simulink model "DR18E_Testpult"  (R2017a)
settings: Solver=ode1  StartTime=0.0  StopTime=Inf  FixedStep=0.001  RelTol=1e-3
PostLoadFcn:
  | , if any(exist('dsrtsu_mdlpostloadfcn', 'file') == [2, 3, 6]), try dsrtsu_mdlpostloadfcn('Execute', bdroot); catch fprintf('Error in PostLoadFcn (dsrtsu_mdlpostloadfcn) for model "%s":\n %s\n', bdroot, lasterr); end, end,
model workspace: external: MAT-File C:\Users\DeltaRacing\Documents\dSPACE\MABX_DR18E\Model\DR18E_MABX_Parameter.mat (data not in the file)
values from neighbouring files (symbols this model uses):
  am = 1/Ts    (= 1)    [DR18E_MABX_Parameter.m]
  bm = K/Ts    (= 0.05)    [DR18E_MABX_Parameter.m]
  cf = 41350    [DR18E_MABX_Parameter.m]
  cr = 41350    [DR18E_MABX_Parameter.m]
  Derating_HV_Battery_Kapa = 1    [DR18E_MABX_Parameter.m]
  Derating_Start_km = 16    [DR18E_MABX_Parameter.m]
  Drive_Mode = 0    [DR18E_MABX_Parameter.m]
  g = 1    [DR18E_MABX_Parameter.m]
  Gas_Modus = 2    [DR18E_MABX_Parameter.m]
  HV_Power_max = 80    [DR18E_MABX_Parameter.m]
  i_Getriebe = 3.3    [DR18E_MABX_Parameter.m]
  i_Lenkgetriebe = 4.32    [DR18E_MABX_Parameter.m]
  K_SET = 1    [DR18E_MABX_Parameter.m]
  Kapazitaet_HV_Battery_kWh = 6.6    [DR18E_MABX_Parameter.m]
  KW_T_Soll = 37    [DR18E_MABX_Parameter.m]
  lf = 1.2    [DR18E_MABX_Parameter.m]
  lr = 1.15    [DR18E_MABX_Parameter.m]
  m = mdriver + mvehicle    (= 310)    [DR18E_MABX_Parameter.m]
  M_max = 150    [DR18E_MABX_Parameter.m]
  Power_Limit_onoff = 0    [DR18E_MABX_Parameter.m]
  Reifenradius = 0.2351    [DR18E_MABX_Parameter.m]
  Strecke_Endu_km = 22    [DR18E_MABX_Parameter.m]
  TC_Decr_Gas = 0.00005    (= 5e-05)    [DR18E_MABX_Parameter.m]
  TC_Derivative = 0.4    [DR18E_MABX_Parameter.m]
  TC_Incr_Gas = 0.005    [DR18E_MABX_Parameter.m]
  TC_On = 0    [DR18E_MABX_Parameter.m]
  TC_Relay_Off = 0.065    [DR18E_MABX_Parameter.m]
  TC_Relay_On = 0.07    [DR18E_MABX_Parameter.m]
  TV_Mode = 2    [DR18E_MABX_Parameter.m]
  TV_On = 0    [DR18E_MABX_Parameter.m]
  TV_Override = 1    [DR18E_MABX_Parameter.m]
  y = 0.8    [DR18E_MABX_Parameter.m]
undefined symbols (not defined in the file or in its folder): D, DiscIntNeverNeededParam, I, K_OL, P
libraries: simulink x288, rtican x100, rtiusbflightreclib x40, rti1401lib_dio_type3 x10, simulink_extras x10, rti1401lib_adc_type4 x8, rti1401lib_II_base x7
(part 23 of 27)

== system DR18E_Testpult/Eingabe Fahrzeug/BMS/Voltage Stack 7-8/Voltage Stack 8 ==
  Timeout[samples] : Inport
  Bus Creator : BusCreator  Inputs=12
  HV_STK8A : rtican/RTICAN Receive (RX)   Reserved1=[]  Reserved2=[]  Reserved3=[]  Reserved4=[]  SfcnMessage=[]  Msg_Struct=[]  BoardTypeNo=[]  BoardNo=[]  ChannelNo=[]  Parameters=[]  DialogFcn=[]  UnitName=[]  Revision=[]  UnitValues=[]  DSProperties=struct('RTI',struct('Version',uint32(5),'BlockType',struct('isSLSource',uint8(1),'isSLSink',uint8(1),'isHWSource',uint8(0),'isHWSink',uint8(0),'isSetup',uint8(0),'isInline',uint8(1),'isNonInline',uint8(0),'isInterrupt',uint8(0),'isChannelwise',uint8(0)),'IOBoardType','RTICAN','UnitType','MESSAGE','Identifier','RX','DialogType','MSVC','BlockSet','RTICAN','SlaveProcessor','CAN'))  RTIBlockInterface=struct('OutputPortsWidth',int32([1 1 1 1 1 1 1]),'OutputPortsActive',[1 1 1 1 1 1 1],'OutputPortsName',{{'Cell_Voltage_85','Cell_Voltage_86','Cell_Voltage_87','Cell_Voltage_88',['RX status'],['RX time'],['RX delta time']}},'OutputPortsDataType',{{'SS_DOUBLE','SS_DOUBLE','SS_DOUBLE','SS_DOUBLE','SS_DOUBLE','SS_DOUBLE','SS_DOUBLE'}},'OutputPortsLabel',{{'Cell_Voltage_85','Cell_Voltage_86','Cell_Voltage_87','Cell_Voltage_88','','',''}},'OutputPortsLabelMode','ON','InputPortsWidth',int32(0),'InputPortsActive',0,'DialogFcn','rtican_message_interface_gui','BlockDisplay',{{'','center'}},'IconTransparency','on','ParameterTunableNames',{{}},'InitLevel',3,'BlockName',struct('Token',{{'HV_STK8A'}}),'SampleTime',{{-1}},'TriggerPort',{{'none'}},'EnablePort',{{'none'}})  RTIBlockParameters=struct('BoardTypeNo',{{1,'OFF',[]}},'BoardNo',{{2,'ON',[1 16]}},'ChannelNo',{{1,'ON',[1 2]}},'Parameters',{{struct('DataFileSupport',struct('DataFileSelectedMaster',1,'DataFileSelectedLocal',1,'DataFileName','c:\users\deltaracing\documents\canoe\dr18e\dbc\dr18e.dbc|','DataFileDate',['16-Feb-2019 13:23:09'],'SelectedFile','..\..\..\canoe\dr18e_test\dr18e\dbc\dr18e.dbc','InterfaceFcn','rtican_dbc_file_parser'),'Options',struct('StatusSelected',1,'TimeSelected',1,'DeltaTimeSelected',1,'BytePortSelected',0,'MessageLengthSelected',0,'TriggerPort',struct('Selected',0,'TriggerType',0),'UserCoding',struct('Selected',0,'InterfaceFile','UserDecodingFile','FcnName','UserDecodeFcn','InportSelected',0,'InportWidth',1,'OutportSelected',0,'OutportWidth',1),'EnablePortSelected',0,'SignalOnPortnameSelected',1,'UseRXService',0),'Message',struct('MsgOnBlocknameSelected',1,'MsgName','HV_STK8A','MsgIdFormat',0,'MsgId',357,'MsgLength',8,'NumSignals',4,'SampleTime',-1,'Signal',struct('SgnName',{'Cell_Voltage_85','Cell_Voltage_86','Cell_Voltage_87','Cell_Voltage_88'},'SgnStartBit',{0,16,32,48},'SgnLength',{16,16,16,16},'ByteLayout',{0,0,0,0},'Factor',{0.001,0.001,0.001,0.001},'Offset',{0,0,0,0},'SgnComment',{'','','',''},'SgnUnit',{'V','V','V','V'},'Min',{0,0,0,0},'Max',{0,0,0,0},'SgnType',{0,0,0,0},'SLDataType',{'SS_DOUBLE','SS_DOUBLE','SS_DOUBLE','SS_DOUBLE'},'DataType',{0,0,0,0},'ModeValue',{-1,-1,-1,-1}),'MsgIdNumFormat',0,'MsgComment',{{''}}),'Version',1.2,'general',struct('isFromLib',0)),'OFF',[]}},'GroupId',{{struct('Group',{{'RTICAN'}},'No',1,'Behavior',{{'NAMECHANGE'}},'BlockType',{{'SINK'}},'NameChangeFlag',0),'OFF',[]}},'SFcnRTICANMessage',{{struct('MsgType','RX','SFcnPortType','Scalar','MsgName','HV_STK8A','MsgIdFormat','STD','MsgId',357,'MsgLength',8,'NumSignals',4,'SampleTime',-1,'Signal',struct('SgnName',{'Cell_Voltage_85','Cell_Voltage_86','Cell_Voltage_87','Cell_Voltage_88'},'SgnStartBit',{0,16,32,48},'SgnLength',{16,16,16,16},'ByteLayout',{['little endian'],['little endian'],['little endian'],['little endian']},'Factor',{0.001,0.001,0.001,0.001},'Offset',{0,0,0,0},'SgnType',{'standard','standard','standard','standard'},'SLDataType',{'SS_DOUBLE','SS_DOUBLE','SS_DOUBLE','SS_DOUBLE'},'DataType',{['unsigned int'],['unsigned int'],['unsigned int'],['unsigned int']},'ModeValue',{-1,-1,-1,-1}),'StatusSelected','yes','TimeSelected','yes','DeltaTimeSelected','yes','BytePortSelected','no','MessageLengthSelected','no','TriggerPort',struct('Selected','no','TriggerType',0),'UserCoding',struct('Selected','no','InterfaceFile','UserDecodingFile','FcnName','UserDecodeFcn','InportSelected','no','InportWidth',1,'OutportSelected','no','OutportWidth',1),'EnablePortSelected','no','UseRXService','no','BoardType','DS1','BoardNo',2,'ControllerNo',1),'OFF',[]}},'TLCFileName',{{'rtican_rx_message','OFF',[]}})  RTISFcnParameters=struct('SFcnRTICANMessage','struct','TLCFileName','char')  RTIBlockParaDefault=struct('BoardTypeNo',4302,'BoardNo',1,'ChannelNo',1,'Parameters',struct('DataFileSupport',struct('DataFileSelectedMaster',0,'DataFileSelectedLocal',0,'DataFileName','','DataFileDate','','SelectedFile',['<no file selected>']),'Options',struct('StatusSelected',1,'TimeSelected',1,'DeltaTimeSelected',1,'BytePortSelected',0,'MessageLengthSelected',0,'TriggerPort',struct('Selected',0,'TriggerType','rising'),'UserCoding',struct('Selected',0,'InterfaceFile','UserDecodingFile','FcnName','UserDecodeFcn','InportSelected',0,'InportWidth',1,'OutportSelected',0,'OutportWidth',1),'EnablePortSelected',0,'SignalOnPortnameSelected',1,'UseRXService',0),'Message',struct('MsgOnBlocknameSelected',0,'MsgName',['RX Message'],'MsgIdFormat',0,'MsgId',100,'MsgLength',8,'NumSignals',1,'SampleTime',-1,'Signal',struct('SgnName',['RX signal'],'SgnStartBit',0,'SgnLength',8,'SgnType',0,'ModeValue',-1,'DataType',0,'SLDataType','SS_DOUBLE','ByteLayout',0,'Factor',1,'Offset',0,'Min',0,'Max',255,'SgnComment',{{}},'SgnUnit',''),'MsgIdNumFormat',0,'MsgComment',{{''}}),'Version',1.2,'general',struct('isFromLib',1)),'GroupId',struct('Group',{{'RTICAN'}},'No',1,'Behavior',{{'NAMECHANGE'}},'BlockType',{{'SINK'}},'NameChangeFlag',0),'SFcnRTICANMessage',struct('MsgType','RX','MsgName',['RX Message'],'MsgIdFormat','STD','MsgId',100,'MsgLength',8,'NumSignals',1,'SampleTime',-1,'Signal',struct('SgnName',['RX signal'],'SgnStartBit',0,'SgnLength',8,'SgnType','standard','ModeValue',-1,'DataType',['unsigned int'],'ByteLayout',['little endian'],'SLDataType','SS_DOUBLE','Factor',1,'Offset',0),'StatusSelected','yes','TimeSelected','yes','DeltaTimeSelected','yes','BytePortSelected','no','MessageLengthSelected','no','EnablePortSelected','no','UserCoding',struct('Selected','no','InterfaceFile','UserDecodingFile','FcnName','UserDecodeFcn','InportSelected','no','InportWidth',1,'OutportSelected','no','OutportWidth',1),'TriggerPort',struct('Selected','no','TriggerType','rising'),'UseRXService','no','BoardType','DS4302','BoardNo',1,'ControllerNo',1,'SFcnPortType','Scalar'),'TLCFileName','rtican_rx_message')
      settings: AttributesFormatString=Group Id: RTICAN1\n  SourceProductName=dSPACE RTI CAN Blockset
  HV_STK8B : rtican/RTICAN Receive (RX)   Reserved1=[]  Reserved2=[]  Reserved3=[]  Reserved4=[]  SfcnMessage=[]  Msg_Struct=[]  BoardTypeNo=[]  BoardNo=[]  ChannelNo=[]  Parameters=[]  DialogFcn=[]  UnitName=[]  Revision=[]  UnitValues=[]  DSProperties=struct('RTI',struct('Version',uint32(5),'BlockType',struct('isSLSource',uint8(1),'isSLSink',uint8(1),'isHWSource',uint8(0),'isHWSink',uint8(0),'isSetup',uint8(0),'isInline',uint8(1),'isNonInline',uint8(0),'isInterrupt',uint8(0),'isChannelwise',uint8(0)),'IOBoardType','RTICAN','UnitType','MESSAGE','Identifier','RX','DialogType','MSVC','BlockSet','RTICAN','SlaveProcessor','CAN'))  RTIBlockInterface=struct('OutputPortsWidth',int32([1 1 1 1 1 1 1]),'OutputPortsActive',[1 1 1 1 1 1 1],'OutputPortsName',{{'Cell_Voltage_89','Cell_Voltage_90','Cell_Voltage_91','Cell_Voltage_92',['RX status'],['RX time'],['RX delta time']}},'OutputPortsDataType',{{'SS_DOUBLE','SS_DOUBLE','SS_DOUBLE','SS_DOUBLE','SS_DOUBLE','SS_DOUBLE','SS_DOUBLE'}},'OutputPortsLabel',{{'Cell_Voltage_89','Cell_Voltage_90','Cell_Voltage_91','Cell_Voltage_92','','',''}},'OutputPortsLabelMode','ON','InputPortsWidth',int32(0),'InputPortsActive',0,'DialogFcn','rtican_message_interface_gui','BlockDisplay',{{'','center'}},'IconTransparency','on','ParameterTunableNames',{{}},'InitLevel',3,'BlockName',struct('Token',{{'HV_STK8B'}}),'SampleTime',{{-1}},'TriggerPort',{{'none'}},'EnablePort',{{'none'}})  RTIBlockParameters=struct('BoardTypeNo',{{1,'OFF',[]}},'BoardNo',{{2,'ON',[1 16]}},'ChannelNo',{{1,'ON',[1 2]}},'Parameters',{{struct('DataFileSupport',struct('DataFileSelectedMaster',1,'DataFileSelectedLocal',1,'DataFileName','c:\users\deltaracing\documents\canoe\dr18e\dbc\dr18e.dbc|','DataFileDate',['16-Feb-2019 13:23:09'],'SelectedFile','..\..\..\canoe\dr18e_test\dr18e\dbc\dr18e.dbc','InterfaceFcn','rtican_dbc_file_parser'),'Options',struct('StatusSelected',1,'TimeSelected',1,'DeltaTimeSelected',1,'BytePortSelected',0,'MessageLengthSelected',0,'TriggerPort',struct('Selected',0,'TriggerType',0),'UserCoding',struct('Selected',0,'InterfaceFile','UserDecodingFile','FcnName','UserDecodeFcn','InportSelected',0,'InportWidth',1,'OutportSelected',0,'OutportWidth',1),'EnablePortSelected',0,'SignalOnPortnameSelected',1,'UseRXService',0),'Message',struct('MsgOnBlocknameSelected',1,'MsgName','HV_STK8B','MsgIdFormat',0,'MsgId',358,'MsgLength',8,'NumSignals',4,'SampleTime',-1,'Signal',struct('SgnName',{'Cell_Voltage_89','Cell_Voltage_90','Cell_Voltage_91','Cell_Voltage_92'},'SgnStartBit',{0,16,32,48},'SgnLength',{16,16,16,16},'ByteLayout',{0,0,0,0},'Factor',{0.001,0.001,0.001,0.001},'Offset',{0,0,0,0},'SgnComment',{'','','',''},'SgnUnit',{'V','V','V','V'},'Min',{0,0,0,0},'Max',{0,0,0,0},'SgnType',{0,0,0,0},'SLDataType',{'SS_DOUBLE','SS_DOUBLE','SS_DOUBLE','SS_DOUBLE'},'DataType',{0,0,0,0},'ModeValue',{-1,-1,-1,-1}),'MsgIdNumFormat',0,'MsgComment',{{''}}),'Version',1.2,'general',struct('isFromLib',0)),'OFF',[]}},'GroupId',{{struct('Group',{{'RTICAN'}},'No',1,'Behavior',{{'NAMECHANGE'}},'BlockType',{{'SINK'}},'NameChangeFlag',0),'OFF',[]}},'SFcnRTICANMessage',{{struct('MsgType','RX','SFcnPortType','Scalar','MsgName','HV_STK8B','MsgIdFormat','STD','MsgId',358,'MsgLength',8,'NumSignals',4,'SampleTime',-1,'Signal',struct('SgnName',{'Cell_Voltage_89','Cell_Voltage_90','Cell_Voltage_91','Cell_Voltage_92'},'SgnStartBit',{0,16,32,48},'SgnLength',{16,16,16,16},'ByteLayout',{['little endian'],['little endian'],['little endian'],['little endian']},'Factor',{0.001,0.001,0.001,0.001},'Offset',{0,0,0,0},'SgnType',{'standard','standard','standard','standard'},'SLDataType',{'SS_DOUBLE','SS_DOUBLE','SS_DOUBLE','SS_DOUBLE'},'DataType',{['unsigned int'],['unsigned int'],['unsigned int'],['unsigned int']},'ModeValue',{-1,-1,-1,-1}),'StatusSelected','yes','TimeSelected','yes','DeltaTimeSelected','yes','BytePortSelected','no','MessageLengthSelected','no','TriggerPort',struct('Selected','no','TriggerType',0),'UserCoding',struct('Selected','no','InterfaceFile','UserDecodingFile','FcnName','UserDecodeFcn','InportSelected','no','InportWidth',1,'OutportSelected','no','OutportWidth',1),'EnablePortSelected','no','UseRXService','no','BoardType','DS1','BoardNo',2,'ControllerNo',1),'OFF',[]}},'TLCFileName',{{'rtican_rx_message','OFF',[]}})  RTISFcnParameters=struct('SFcnRTICANMessage','struct','TLCFileName','char')  RTIBlockParaDefault=struct('BoardTypeNo',4302,'BoardNo',1,'ChannelNo',1,'Parameters',struct('DataFileSupport',struct('DataFileSelectedMaster',0,'DataFileSelectedLocal',0,'DataFileName','','DataFileDate','','SelectedFile',['<no file selected>']),'Options',struct('StatusSelected',1,'TimeSelected',1,'DeltaTimeSelected',1,'BytePortSelected',0,'MessageLengthSelected',0,'TriggerPort',struct('Selected',0,'TriggerType','rising'),'UserCoding',struct('Selected',0,'InterfaceFile','UserDecodingFile','FcnName','UserDecodeFcn','InportSelected',0,'InportWidth',1,'OutportSelected',0,'OutportWidth',1),'EnablePortSelected',0,'SignalOnPortnameSelected',1,'UseRXService',0),'Message',struct('MsgOnBlocknameSelected',0,'MsgName',['RX Message'],'MsgIdFormat',0,'MsgId',100,'MsgLength',8,'NumSignals',1,'SampleTime',-1,'Signal',struct('SgnName',['RX signal'],'SgnStartBit',0,'SgnLength',8,'SgnType',0,'ModeValue',-1,'DataType',0,'SLDataType','SS_DOUBLE','ByteLayout',0,'Factor',1,'Offset',0,'Min',0,'Max',255,'SgnComment',{{}},'SgnUnit',''),'MsgIdNumFormat',0,'MsgComment',{{''}}),'Version',1.2,'general',struct('isFromLib',1)),'GroupId',struct('Group',{{'RTICAN'}},'No',1,'Behavior',{{'NAMECHANGE'}},'BlockType',{{'SINK'}},'NameChangeFlag',0),'SFcnRTICANMessage',struct('MsgType','RX','MsgName',['RX Message'],'MsgIdFormat','STD','MsgId',100,'MsgLength',8,'NumSignals',1,'SampleTime',-1,'Signal',struct('SgnName',['RX signal'],'SgnStartBit',0,'SgnLength',8,'SgnType','standard','ModeValue',-1,'DataType',['unsigned int'],'ByteLayout',['little endian'],'SLDataType','SS_DOUBLE','Factor',1,'Offset',0),'StatusSelected','yes','TimeSelected','yes','DeltaTimeSelected','yes','BytePortSelected','no','MessageLengthSelected','no','EnablePortSelected','no','UserCoding',struct('Selected','no','InterfaceFile','UserDecodingFile','FcnName','UserDecodeFcn','InportSelected','no','InportWidth',1,'OutportSelected','no','OutportWidth',1),'TriggerPort',struct('Selected','no','TriggerType','rising'),'UseRXService','no','BoardType','DS4302','BoardNo',1,'ControllerNo',1,'SFcnPortType','Scalar'),'TLCFileName','rtican_rx_message')
      settings: AttributesFormatString=Group Id: RTICAN1\n  SourceProductName=dSPACE RTI CAN Blockset
  HV_STK8C : rtican/RTICAN Receive (RX)   Reserved1=[]  Reserved2=[]  Reserved3=[]  Reserved4=[]  SfcnMessage=[]  Msg_Struct=[]  BoardTypeNo=[]  BoardNo=[]  ChannelNo=[]  Parameters=[]  DialogFcn=[]  UnitName=[]  Revision=[]  UnitValues=[]  DSProperties=struct('RTI',struct('Version',uint32(5),'BlockType',struct('isSLSource',uint8(1),'isSLSink',uint8(1),'isHWSource',uint8(0),'isHWSink',uint8(0),'isSetup',uint8(0),'isInline',uint8(1),'isNonInline',uint8(0),'isInterrupt',uint8(0),'isChannelwise',uint8(0)),'IOBoardType','RTICAN','UnitType','MESSAGE','Identifier','RX','DialogType','MSVC','BlockSet','RTICAN','SlaveProcessor','CAN'))  RTIBlockInterface=struct('OutputPortsWidth',int32([1 1 1 1 1 1 1]),'OutputPortsActive',[1 1 1 1 1 1 1],'OutputPortsName',{{'Cell_Voltage_93','Cell_Voltage_94','Cell_Voltage_95','Cell_Voltage_96',['RX status'],['RX time'],['RX delta time']}},'OutputPortsDataType',{{'SS_DOUBLE','SS_DOUBLE','SS_DOUBLE','SS_DOUBLE','SS_DOUBLE','SS_DOUBLE','SS_DOUBLE'}},'OutputPortsLabel',{{'Cell_Voltage_93','Cell_Voltage_94','Cell_Voltage_95','Cell_Voltage_96','','',''}},'OutputPortsLabelMode','ON','InputPortsWidth',int32(0),'InputPortsActive',0,'DialogFcn','rtican_message_interface_gui','BlockDisplay',{{'','center'}},'IconTransparency','on','ParameterTunableNames',{{}},'InitLevel',3,'BlockName',struct('Token',{{'HV_STK8C'}}),'SampleTime',{{-1}},'TriggerPort',{{'none'}},'EnablePort',{{'none'}})  RTIBlockParameters=struct('BoardTypeNo',{{1,'OFF',[]}},'BoardNo',{{2,'ON',[1 16]}},'ChannelNo',{{1,'ON',[1 2]}},'Parameters',{{struct('DataFileSupport',struct('DataFileSelectedMaster',1,'DataFileSelectedLocal',1,'DataFileName','c:\users\deltaracing\documents\canoe\dr18e\dbc\dr18e.dbc|','DataFileDate',['16-Feb-2019 13:23:09'],'SelectedFile','..\..\..\canoe\dr18e_test\dr18e\dbc\dr18e.dbc','InterfaceFcn','rtican_dbc_file_parser'),'Options',struct('StatusSelected',1,'TimeSelected',1,'DeltaTimeSelected',1,'BytePortSelected',0,'MessageLengthSelected',0,'TriggerPort',struct('Selected',0,'TriggerType',0),'UserCoding',struct('Selected',0,'InterfaceFile','UserDecodingFile','FcnName','UserDecodeFcn','InportSelected',0,'InportWidth',1,'OutportSelected',0,'OutportWidth',1),'EnablePortSelected',0,'SignalOnPortnameSelected',1,'UseRXService',0),'Message',struct('MsgOnBlocknameSelected',1,'MsgName','HV_STK8C','MsgIdFormat',0,'MsgId',359,'MsgLength',8,'NumSignals',4,'SampleTime',-1,'Signal',struct('SgnName',{'Cell_Voltage_93','Cell_Voltage_94','Cell_Voltage_95','Cell_Voltage_96'},'SgnStartBit',{0,16,32,48},'SgnLength',{16,16,16,16},'ByteLayout',{0,0,0,0},'Factor',{0.001,0.001,0.001,0.001},'Offset',{0,0,0,0},'SgnComment',{'','','',''},'SgnUnit',{'V','V','V','V'},'Min',{0,0,0,0},'Max',{0,0,0,0},'SgnType',{0,0,0,0},'SLDataType',{'SS_DOUBLE','SS_DOUBLE','SS_DOUBLE','SS_DOUBLE'},'DataType',{0,0,0,0},'ModeValue',{-1,-1,-1,-1}),'MsgIdNumFormat',0,'MsgComment',{{''}}),'Version',1.2,'general',struct('isFromLib',0)),'OFF',[]}},'GroupId',{{struct('Group',{{'RTICAN'}},'No',1,'Behavior',{{'NAMECHANGE'}},'BlockType',{{'SINK'}},'NameChangeFlag',0),'OFF',[]}},'SFcnRTICANMessage',{{struct('MsgType','RX','SFcnPortType','Scalar','MsgName','HV_STK8C','MsgIdFormat','STD','MsgId',359,'MsgLength',8,'NumSignals',4,'SampleTime',-1,'Signal',struct('SgnName',{'Cell_Voltage_93','Cell_Voltage_94','Cell_Voltage_95','Cell_Voltage_96'},'SgnStartBit',{0,16,32,48},'SgnLength',{16,16,16,16},'ByteLayout',{['little endian'],['little endian'],['little endian'],['little endian']},'Factor',{0.001,0.001,0.001,0.001},'Offset',{0,0,0,0},'SgnType',{'standard','standard','standard','standard'},'SLDataType',{'SS_DOUBLE','SS_DOUBLE','SS_DOUBLE','SS_DOUBLE'},'DataType',{['unsigned int'],['unsigned int'],['unsigned int'],['unsigned int']},'ModeValue',{-1,-1,-1,-1}),'StatusSelected','yes','TimeSelected','yes','DeltaTimeSelected','yes','BytePortSelected','no','MessageLengthSelected','no','TriggerPort',struct('Selected','no','TriggerType',0),'UserCoding',struct('Selected','no','InterfaceFile','UserDecodingFile','FcnName','UserDecodeFcn','InportSelected','no','InportWidth',1,'OutportSelected','no','OutportWidth',1),'EnablePortSelected','no','UseRXService','no','BoardType','DS1','BoardNo',2,'ControllerNo',1),'OFF',[]}},'TLCFileName',{{'rtican_rx_message','OFF',[]}})  RTISFcnParameters=struct('SFcnRTICANMessage','struct','TLCFileName','char')  RTIBlockParaDefault=struct('BoardTypeNo',4302,'BoardNo',1,'ChannelNo',1,'Parameters',struct('DataFileSupport',struct('DataFileSelectedMaster',0,'DataFileSelectedLocal',0,'DataFileName','','DataFileDate','','SelectedFile',['<no file selected>']),'Options',struct('StatusSelected',1,'TimeSelected',1,'DeltaTimeSelected',1,'BytePortSelected',0,'MessageLengthSelected',0,'TriggerPort',struct('Selected',0,'TriggerType','rising'),'UserCoding',struct('Selected',0,'InterfaceFile','UserDecodingFile','FcnName','UserDecodeFcn','InportSelected',0,'InportWidth',1,'OutportSelected',0,'OutportWidth',1),'EnablePortSelected',0,'SignalOnPortnameSelected',1,'UseRXService',0),'Message',struct('MsgOnBlocknameSelected',0,'MsgName',['RX Message'],'MsgIdFormat',0,'MsgId',100,'MsgLength',8,'NumSignals',1,'SampleTime',-1,'Signal',struct('SgnName',['RX signal'],'SgnStartBit',0,'SgnLength',8,'SgnType',0,'ModeValue',-1,'DataType',0,'SLDataType','SS_DOUBLE','ByteLayout',0,'Factor',1,'Offset',0,'Min',0,'Max',255,'SgnComment',{{}},'SgnUnit',''),'MsgIdNumFormat',0,'MsgComment',{{''}}),'Version',1.2,'general',struct('isFromLib',1)),'GroupId',struct('Group',{{'RTICAN'}},'No',1,'Behavior',{{'NAMECHANGE'}},'BlockType',{{'SINK'}},'NameChangeFlag',0),'SFcnRTICANMessage',struct('MsgType','RX','MsgName',['RX Message'],'MsgIdFormat','STD','MsgId',100,'MsgLength',8,'NumSignals',1,'SampleTime',-1,'Signal',struct('SgnName',['RX signal'],'SgnStartBit',0,'SgnLength',8,'SgnType','standard','ModeValue',-1,'DataType',['unsigned int'],'ByteLayout',['little endian'],'SLDataType','SS_DOUBLE','Factor',1,'Offset',0),'StatusSelected','yes','TimeSelected','yes','DeltaTimeSelected','yes','BytePortSelected','no','MessageLengthSelected','no','EnablePortSelected','no','UserCoding',struct('Selected','no','InterfaceFile','UserDecodingFile','FcnName','UserDecodeFcn','InportSelected','no','InportWidth',1,'OutportSelected','no','OutportWidth',1),'TriggerPort',struct('Selected','no','TriggerType','rising'),'UseRXService','no','BoardType','DS4302','BoardNo',1,'ControllerNo',1,'SFcnPortType','Scalar'),'TLCFileName','rtican_rx_message')
      settings: AttributesFormatString=Group Id: RTICAN1\n  SourceProductName=dSPACE RTI CAN Blockset
  Logical Operator : Logic  Operator=OR  Inputs=3  AllPortsSameDT=off  OutDataTypeStr=boolean
  RX Timeout Detection : Subsystem
  RX Timeout Detection1 : Subsystem
  RX Timeout Detection2 : Subsystem
  Cell73-84 : Outport
  TimeoutError : Outport  Port=2
  wires:
  HV_STK8B/5 -> RX Timeout Detection/1(RX status)
  HV_STK8C/5 -> RX Timeout Detection2/1(RX status)
  Bus Creator/1 -> Cell73-84/1  "Cell73-84"
  HV_STK8A/5 -> RX Timeout Detection1/1(RX status)
  RX Timeout Detection2/1(RX Timeout Error) -> Logical Operator/3
  RX Timeout Detection/1(RX Timeout Error) -> Logical Operator/2  "RX Timeout Error"
  RX Timeout Detection1/1(RX Timeout Error) -> Logical Operator/1
  Logical Operator/1 -> TimeoutError/1
  Timeout[samples]/1 -> RX Timeout Detection1/2(Timeout (n Samples)), RX Timeout Detection/2(Timeout (n Samples)), RX Timeout Detection2/2(Timeout (n Samples))
  HV_STK8A/1 -> Bus Creator/1  "Cell_Voltage_85"
  HV_STK8A/2 -> Bus Creator/2  "Cell_Voltage_86"
  HV_STK8A/3 -> Bus Creator/3  "Cell_Voltage_87"
  HV_STK8A/4 -> Bus Creator/4  "Cell_Voltage_88"
  HV_STK8B/1 -> Bus Creator/5  "Cell_Voltage_89"
  HV_STK8B/2 -> Bus Creator/6  "Cell_Voltage_90"
  HV_STK8B/3 -> Bus Creator/7  "Cell_Voltage_91"
  HV_STK8B/4 -> Bus Creator/8  "Cell_Voltage_92"
  HV_STK8C/1 -> Bus Creator/9  "Cell_Voltage_93"
  HV_STK8C/2 -> Bus Creator/10  "Cell_Voltage_94"
  HV_STK8C/3 -> Bus Creator/11  "Cell_Voltage_95"
  HV_STK8C/4 -> Bus Creator/12  "Cell_Voltage_96"

== system DR18E_Testpult/Eingabe Fahrzeug/Gyro/RX Timeout Detection/Triggered Subsystem ==
  TXStatus : Inport
  Timeout : Inport  Port=2
  Constant : Constant
  Constant1 : Constant  Value=0
  Constant2 : Constant
  Constant3 : Constant  Value=0
  Delay : Delay  DelayLength=1  InitialCondition=0
  Relational Operator : RelationalOperator  Operator=>  OutDataTypeStr=boolean  RndMeth=Nearest
  Sum : Sum  Inputs=|++
  Switch : Switch  Criteria=u2 > Threshold
  Switch1 : Switch  Criteria=u2 > Threshold
  Rampe : Outport
  RX Timeout Error : Outport  Port=2
  wires:
  TXStatus/1 -> Switch/2
  Delay/1 -> Sum/2
  Constant/1 -> Sum/1
  Sum/1 -> Switch/3
  Switch/1 -> Delay/1, Relational Operator/1, Rampe/1
  Constant1/1 -> Switch/1
  Constant2/1 -> Switch1/1
  Constant3/1 -> Switch1/3
  Switch1/1 -> RX Timeout Error/1
  Relational Operator/1 -> Switch1/2
  Timeout/1 -> Relational Operator/2

== system DR18E_Testpult/Eingabe Fahrzeug/Inverter Feedback Messages/Istwerte Umrichter 1 empfangen /Drehzahl ==
  CAN Value : Inport
  M_Mot : Inport  Port=2
  Action Port : ActionPort  ActionType=case
  2*pi / 60 : Gain  Gain=1.8*6.283185 / 60
  Constant1 : Constant
  Data Type Conversion : DataTypeConversion  OutDataTypeStr=int16
  Data Type Conversion1 : DataTypeConversion  OutDataTypeStr=double
  PT1 Discrete2 : Subsystem
  Product : Product
  Skalierung Drehzahl : Subsystem  TreatAsAtomicUnit=on
  TFilterDrehzahl : Constant  Value=0.01
  Drehzahl in 1/min U1 : Outport
  Motorleistung in W U1 : Outport  Port=2
  wires:
  CAN Value/1 -> Data Type Conversion/1
  Skalierung Drehzahl/1(Out1) -> PT1 Discrete2/1(u)
  Data Type Conversion/1 -> Data Type Conversion1/1
  Product/1 -> 2*pi / 60/1
  M_Mot/1 -> Product/2
  2*pi / 60/1 -> Motorleistung in W U1/1
  Constant1/1 -> PT1 Discrete2/2(K)
  TFilterDrehzahl/1 -> PT1 Discrete2/3(T)
  PT1 Discrete2/1(y) -> Drehzahl in 1/min U1/1, Product/1
  Data Type Conversion1/1 -> Skalierung Drehzahl/1(In1)

== system DR18E_Testpult/Eingabe Fahrzeug/Inverter Feedback Messages/Istwerte Umrichter 1 empfangen /FlightRecorder1 ==
  In1 : Inport
  Data Type Conversion : DataTypeConversion
  Gain : Gain
  USB_FLIGHT_REC_BL1 : rtiusbflightreclib/USB_FLIGHT_REC_BL1  VarName=UDC_HV  DataType=Single  SampleTime=-1  TLCFileName=rtiusbflightrecwrite  Reserved1=[]  Reserved2=[]  Reserved3=[]  Reserved4=[]  DSProperties=struct('RTI',struct('Version',uint32(3),'BlockType',struct('isSLSource',uint8(0),'isSLSink',uint8(1),'isHWSource',uint8(0),'isHWSink',uint8(0),'isSetup',uint8(0),'isInline',uint8(1),'isNonInline',uint8(0),'isInterrupt',uint8(0),'isChannelwise',uint8(0)),'IOBoardType',{{'DSUSB','FLIGHTREC'}},'UnitType','FLIGHTREC','Identifier','WRITE','DialogType','SL','BlockSet','RTIUSBFLIGHTREC','SlaveProcessor','NONE'))  RTIBlockInterface=struct('InputPortsActive',1,'InputPortsWidth',int32(1),'InputPortsDataType',{{'SS_SINGLE'}},'BlockDisplay',{{['Write to\nUSB Flight Recorder'],'center'}},'IconTransparency','off','InitLevel',3,'BlockName',struct('Token',{{'USB_FLIGHT_REC_BL1'}}),'MaskDescription',['Write input to the Flight Recorder. Recorded data can be referenced by the specified variable.'],'SampleTime',{{-1}})  RTIBlockParameters=struct('VarName',{{'UDC_HV','OFF',[]}},'DataType',{{'Single','OFF',[]}},'SampleTime',{{-1,'OFF',[]}},'TLCFileName',{{'rtiusbflightrecwrite','OFF',[]}})  RTISFcnParameters=struct('VarName','char','DataType','char','SampleTime','double','TLCFileName','char')  RTIBlockParaDefault=struct('VarName','Var1','DataType','Single','SampleTime',-1,'TLCFileName','rtiusbflightrecwrite')
      settings: SourceProductName=dSPACE RTI USB Flight Rec Blockset
  wires:
  Data Type Conversion/1 -> USB_FLIGHT_REC_BL1/1
  In1/1 -> Gain/1
  Gain/1 -> Data Type Conversion/1

== system DR18E_Testpult/Eingabe Fahrzeug/Inverter Feedback Messages/Istwerte Umrichter 1 empfangen /FlightRecorder2 ==
  In1 : Inport
  Data Type Conversion : DataTypeConversion
  Gain : Gain
  USB_FLIGHT_REC_BL1 : rtiusbflightreclib/USB_FLIGHT_REC_BL1  VarName=Inverter1Temp  DataType=Single  SampleTime=-1  TLCFileName=rtiusbflightrecwrite  Reserved1=[]  Reserved2=[]  Reserved3=[]  Reserved4=[]  DSProperties=struct('RTI',struct('Version',uint32(3),'BlockType',struct('isSLSource',uint8(0),'isSLSink',uint8(1),'isHWSource',uint8(0),'isHWSink',uint8(0),'isSetup',uint8(0),'isInline',uint8(1),'isNonInline',uint8(0),'isInterrupt',uint8(0),'isChannelwise',uint8(0)),'IOBoardType',{{'DSUSB','FLIGHTREC'}},'UnitType','FLIGHTREC','Identifier','WRITE','DialogType','SL','BlockSet','RTIUSBFLIGHTREC','SlaveProcessor','NONE'))  RTIBlockInterface=struct('InputPortsActive',1,'InputPortsWidth',int32(1),'InputPortsDataType',{{'SS_SINGLE'}},'BlockDisplay',{{['Write to\nUSB Flight Recorder'],'center'}},'IconTransparency','off','InitLevel',3,'BlockName',struct('Token',{{'USB_FLIGHT_REC_BL1'}}),'MaskDescription',['Write input to the Flight Recorder. Recorded data can be referenced by the specified variable.'],'SampleTime',{{-1}})  RTIBlockParameters=struct('VarName',{{'Inverter1Temp','OFF',[]}},'DataType',{{'Single','OFF',[]}},'SampleTime',{{-1,'OFF',[]}},'TLCFileName',{{'rtiusbflightrecwrite','OFF',[]}})  RTISFcnParameters=struct('VarName','char','DataType','char','SampleTime','double','TLCFileName','char')  RTIBlockParaDefault=struct('VarName','Var1','DataType','Single','SampleTime',-1,'TLCFileName','rtiusbflightrecwrite')
      settings: SourceProductName=dSPACE RTI USB Flight Rec Blockset
  wires:
  Data Type Conversion/1 -> USB_FLIGHT_REC_BL1/1
  In1/1 -> Gain/1
  Gain/1 -> Data Type Conversion/1

== system DR18E_Testpult/Eingabe Fahrzeug/Inverter Feedback Messages/Istwerte Umrichter 1 empfangen /FlightRecorder3 ==
  In1 : Inport
  Data Type Conversion : DataTypeConversion
  Gain : Gain
  USB_FLIGHT_REC_BL1 : rtiusbflightreclib/USB_FLIGHT_REC_BL1  VarName=MMotL_ist  DataType=Single  SampleTime=-1  TLCFileName=rtiusbflightrecwrite  Reserved1=[]  Reserved2=[]  Reserved3=[]  Reserved4=[]  DSProperties=struct('RTI',struct('Version',uint32(3),'BlockType',struct('isSLSource',uint8(0),'isSLSink',uint8(1),'isHWSource',uint8(0),'isHWSink',uint8(0),'isSetup',uint8(0),'isInline',uint8(1),'isNonInline',uint8(0),'isInterrupt',uint8(0),'isChannelwise',uint8(0)),'IOBoardType',{{'DSUSB','FLIGHTREC'}},'UnitType','FLIGHTREC','Identifier','WRITE','DialogType','SL','BlockSet','RTIUSBFLIGHTREC','SlaveProcessor','NONE'))  RTIBlockInterface=struct('InputPortsActive',1,'InputPortsWidth',int32(1),'InputPortsDataType',{{'SS_SINGLE'}},'BlockDisplay',{{['Write to\nUSB Flight Recorder'],'center'}},'IconTransparency','off','InitLevel',3,'BlockName',struct('Token',{{'USB_FLIGHT_REC_BL1'}}),'MaskDescription',['Write input to the Flight Recorder. Recorded data can be referenced by the specified variable.'],'SampleTime',{{-1}})  RTIBlockParameters=struct('VarName',{{'MMotL_ist','OFF',[]}},'DataType',{{'Single','OFF',[]}},'SampleTime',{{-1,'OFF',[]}},'TLCFileName',{{'rtiusbflightrecwrite','OFF',[]}})  RTISFcnParameters=struct('VarName','char','DataType','char','SampleTime','double','TLCFileName','char')  RTIBlockParaDefault=struct('VarName','Var1','DataType','Single','SampleTime',-1,'TLCFileName','rtiusbflightrecwrite')
      settings: SourceProductName=dSPACE RTI USB Flight Rec Blockset
  wires:
  Data Type Conversion/1 -> USB_FLIGHT_REC_BL1/1
  In1/1 -> Gain/1
  Gain/1 -> Data Type Conversion/1

== system DR18E_Testpult/Eingabe Fahrzeug/Inverter Feedback Messages/Istwerte Umrichter 1 empfangen /FlightRecorder4 ==
  In1 : Inport
  Data Type Conversion : DataTypeConversion
  Gain : Gain
  USB_FLIGHT_REC_BL1 : rtiusbflightreclib/USB_FLIGHT_REC_BL1  VarName=MotorLTemp  DataType=Single  SampleTime=-1  TLCFileName=rtiusbflightrecwrite  Reserved1=[]  Reserved2=[]  Reserved3=[]  Reserved4=[]  DSProperties=struct('RTI',struct('Version',uint32(3),'BlockType',struct('isSLSource',uint8(0),'isSLSink',uint8(1),'isHWSource',uint8(0),'isHWSink',uint8(0),'isSetup',uint8(0),'isInline',uint8(1),'isNonInline',uint8(0),'isInterrupt',uint8(0),'isChannelwise',uint8(0)),'IOBoardType',{{'DSUSB','FLIGHTREC'}},'UnitType','FLIGHTREC','Identifier','WRITE','DialogType','SL','BlockSet','RTIUSBFLIGHTREC','SlaveProcessor','NONE'))  RTIBlockInterface=struct('InputPortsActive',1,'InputPortsWidth',int32(1),'InputPortsDataType',{{'SS_SINGLE'}},'BlockDisplay',{{['Write to\nUSB Flight Recorder'],'center'}},'IconTransparency','off','InitLevel',3,'BlockName',struct('Token',{{'USB_FLIGHT_REC_BL1'}}),'MaskDescription',['Write input to the Flight Recorder. Recorded data can be referenced by the specified variable.'],'SampleTime',{{-1}})  RTIBlockParameters=struct('VarName',{{'MotorLTemp','OFF',[]}},'DataType',{{'Single','OFF',[]}},'SampleTime',{{-1,'OFF',[]}},'TLCFileName',{{'rtiusbflightrecwrite','OFF',[]}})  RTISFcnParameters=struct('VarName','char','DataType','char','SampleTime','double','TLCFileName','char')  RTIBlockParaDefault=struct('VarName','Var1','DataType','Single','SampleTime',-1,'TLCFileName','rtiusbflightrecwrite')
      settings: SourceProductName=dSPACE RTI USB Flight Rec Blockset
  wires:
  Data Type Conversion/1 -> USB_FLIGHT_REC_BL1/1
  In1/1 -> Gain/1
  Gain/1 -> Data Type Conversion/1

== system DR18E_Testpult/Eingabe Fahrzeug/Inverter Feedback Messages/Istwerte Umrichter 1 empfangen /Inverter_Temp ==
  In1 : Inport
  Action Port : ActionPort  ActionType=case
  "BAMOCAR PG D3 Manual S. 48 " : Lookup_n-D  NumberOfTableDimensions=1  BreakpointsForDimension1=[17151,17400,17688,18017,18387,18797,19247,19733,20250,20793,21357,21933,22515,23097,23671,24232,24775,25296,25792,26261,26702]  Table=[0,5,10,15,20,25,30,35,40,45,50,55,60,65,70,75,80,85,90,95,100]  RndMeth=Simplest  InputSameDT=on
  Inverter_Temp : Outport
  wires:
  In1/1 -> "BAMOCAR PG D3 Manual S. 48 "/1  "Wert"
  "BAMOCAR PG D3 Manual S. 48 "/1 -> Inverter_Temp/1

== system DR18E_Testpult/Eingabe Fahrzeug/Inverter Feedback Messages/Istwerte Umrichter 1 empfangen /Motortemperatur ==
  In1 : Inport
  Action Port : ActionPort  ActionType=case
  Constant2 : Constant  Value=37175
  Divide : Product  Inputs=*/
  Gain : Gain  Gain=4700
  Subtract : Sum  Inputs=+-
  Temp. corresponding resistance : Lookup_n-D  NumberOfTableDimensions=1  BreakpointsForDimension1=[1030,1135,1247,1367,1495,1630,1772,1922,2000,2080,2245,2417,2597,2785,2980,3182,3392,3607,3817,3915,4008,4166,4280]  IndexSearchMethod=Linear search  Table=[-50,-40,-30,-20,-10,0,10,20,25,30,40,50,60,70,80,90,100,110,120,125,130,140,150]  RndMeth=Simplest  InputSameDT=on
  Motor1_Temp : Outport
  "Motor1_Temp_Raw " : Outport  Port=2
  wires:
  Gain/1 -> Divide/1
  Subtract/1 -> Divide/2  "RawWert2_Motor1"
  Constant2/1 -> Subtract/1
  In1/1 -> Subtract/2, Gain/1  "Wert"
  Divide/1 -> "Motor1_Temp_Raw "/1, Temp. corresponding resistance/1
  Temp. corresponding resistance/1 -> Motor1_Temp/1

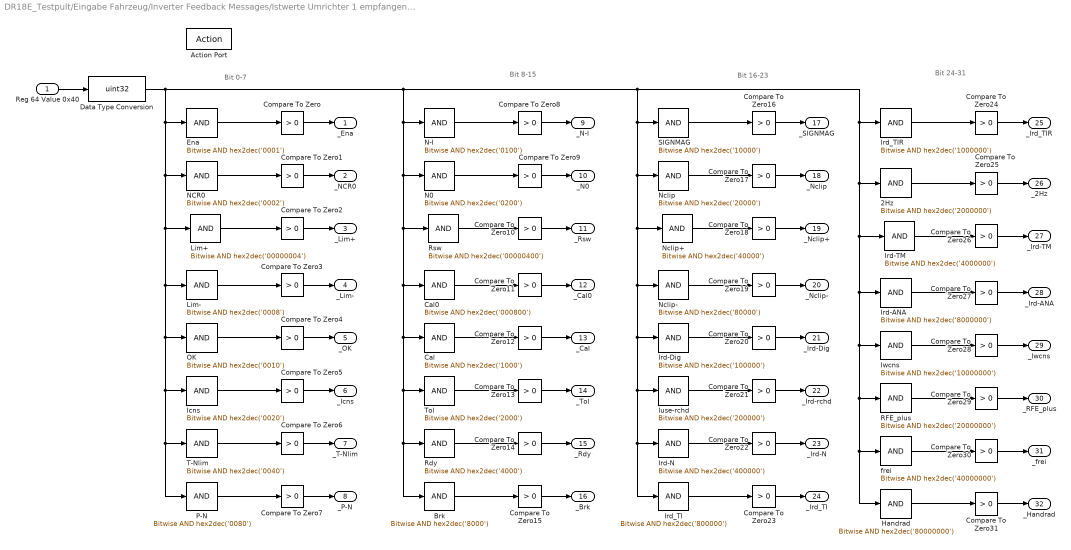
== system DR18E_Testpult/Eingabe Fahrzeug/Inverter Feedback Messages/Istwerte Umrichter 1 empfangen /Red ID 64: Status Register Auswertung ==
  note: Bit 24-31
  note: Bit 16-23
  note: Bit 8-15
  note: Bit 0-7
  Reg 64 Value 0x40 : Inport
  Action Port : ActionPort  ActionType=case
  2Hz : simulink/Logic and Bit Operations/Bitwise Operator  logicop=AND  UseBitMask=on  BitMask=hex2dec('2000000')  BitMaskRealWorld=Stored Integer
  Brk : simulink/Logic and Bit Operations/Bitwise Operator  logicop=AND  UseBitMask=on  BitMask=hex2dec('8000')  BitMaskRealWorld=Stored Integer
  Cal : simulink/Logic and Bit Operations/Bitwise Operator  logicop=AND  UseBitMask=on  BitMask=hex2dec('1000')  BitMaskRealWorld=Stored Integer
  Cal0 : simulink/Logic and Bit Operations/Bitwise Operator  logicop=AND  UseBitMask=on  BitMask=hex2dec('000800')  BitMaskRealWorld=Stored Integer
  Compare To Zero{,1..31} (32 alike) : simulink/Logic and Bit Operations/Compare To Zero  relop=>  OutDataTypeStr=boolean
  Data Type Conversion : DataTypeConversion  OutDataTypeStr=uint32
  Ena : simulink/Logic and Bit Operations/Bitwise Operator  logicop=AND  UseBitMask=on  BitMask=hex2dec('0001')  BitMaskRealWorld=Stored Integer
  Handrad : simulink/Logic and Bit Operations/Bitwise Operator  logicop=AND  UseBitMask=on  BitMask=hex2dec('80000000')  BitMaskRealWorld=Stored Integer
  Icns : simulink/Logic and Bit Operations/Bitwise Operator  logicop=AND  UseBitMask=on  BitMask=hex2dec('0020')  BitMaskRealWorld=Stored Integer
  Ird-ANA : simulink/Logic and Bit Operations/Bitwise Operator  logicop=AND  UseBitMask=on  BitMask=hex2dec('8000000')  BitMaskRealWorld=Stored Integer
  Ird-Dig : simulink/Logic and Bit Operations/Bitwise Operator  logicop=AND  UseBitMask=on  BitMask=hex2dec('100000')  BitMaskRealWorld=Stored Integer
  Ird-N : simulink/Logic and Bit Operations/Bitwise Operator  logicop=AND  UseBitMask=on  BitMask=hex2dec('400000')  BitMaskRealWorld=Stored Integer
  Ird-TM : simulink/Logic and Bit Operations/Bitwise Operator  logicop=AND  UseBitMask=on  BitMask=hex2dec('4000000')  BitMaskRealWorld=Stored Integer
  Ird_TI : simulink/Logic and Bit Operations/Bitwise Operator  logicop=AND  UseBitMask=on  BitMask=hex2dec('800000')  BitMaskRealWorld=Stored Integer
  Ird_TIR : simulink/Logic and Bit Operations/Bitwise Operator  logicop=AND  UseBitMask=on  BitMask=hex2dec('1000000')  BitMaskRealWorld=Stored Integer
  Iuse-rchd : simulink/Logic and Bit Operations/Bitwise Operator  logicop=AND  UseBitMask=on  BitMask=hex2dec('200000')  BitMaskRealWorld=Stored Integer
  Iwcns : simulink/Logic and Bit Operations/Bitwise Operator  logicop=AND  UseBitMask=on  BitMask=hex2dec('10000000')  BitMaskRealWorld=Stored Integer
  Lim+ : simulink/Logic and Bit Operations/Bitwise Operator  logicop=AND  UseBitMask=on  BitMask=hex2dec('00000004')  BitMaskRealWorld=Stored Integer
  Lim- : simulink/Logic and Bit Operations/Bitwise Operator  logicop=AND  UseBitMask=on  BitMask=hex2dec('0008')  BitMaskRealWorld=Stored Integer
  N-I : simulink/Logic and Bit Operations/Bitwise Operator  logicop=AND  UseBitMask=on  BitMask=hex2dec('0100')  BitMaskRealWorld=Stored Integer
  N0 : simulink/Logic and Bit Operations/Bitwise Operator  logicop=AND  UseBitMask=on  BitMask=hex2dec('0200')  BitMaskRealWorld=Stored Integer
  NCR0 : simulink/Logic and Bit Operations/Bitwise Operator  logicop=AND  UseBitMask=on  BitMask=hex2dec('0002')  BitMaskRealWorld=Stored Integer
  Nclip : simulink/Logic and Bit Operations/Bitwise Operator  logicop=AND  UseBitMask=on  BitMask=hex2dec('20000')  BitMaskRealWorld=Stored Integer
  Nclip+ : simulink/Logic and Bit Operations/Bitwise Operator  logicop=AND  UseBitMask=on  BitMask=hex2dec('40000')  BitMaskRealWorld=Stored Integer
  Nclip- : simulink/Logic and Bit Operations/Bitwise Operator  logicop=AND  UseBitMask=on  BitMask=hex2dec('80000')  BitMaskRealWorld=Stored Integer
  OK : simulink/Logic and Bit Operations/Bitwise Operator  logicop=AND  UseBitMask=on  BitMask=hex2dec('0010')  BitMaskRealWorld=Stored Integer
  P-N : simulink/Logic and Bit Operations/Bitwise Operator  logicop=AND  UseBitMask=on  BitMask=hex2dec('0080')  BitMaskRealWorld=Stored Integer
  RFE_plus : simulink/Logic and Bit Operations/Bitwise Operator  logicop=AND  UseBitMask=on  BitMask=hex2dec('20000000')  BitMaskRealWorld=Stored Integer
  Rdy : simulink/Logic and Bit Operations/Bitwise Operator  logicop=AND  UseBitMask=on  BitMask=hex2dec('4000')  BitMaskRealWorld=Stored Integer
  Rsw : simulink/Logic and Bit Operations/Bitwise Operator  logicop=AND  UseBitMask=on  BitMask=hex2dec('00000400')  BitMaskRealWorld=Stored Integer
  SIGNMAG : simulink/Logic and Bit Operations/Bitwise Operator  logicop=AND  UseBitMask=on  BitMask=hex2dec('10000')  BitMaskRealWorld=Stored Integer
  T-Nlim : simulink/Logic and Bit Operations/Bitwise Operator  logicop=AND  UseBitMask=on  BitMask=hex2dec('0040')  BitMaskRealWorld=Stored Integer
  Tol : simulink/Logic and Bit Operations/Bitwise Operator  logicop=AND  UseBitMask=on  BitMask=hex2dec('2000')  BitMaskRealWorld=Stored Integer
  frei : simulink/Logic and Bit Operations/Bitwise Operator  logicop=AND  UseBitMask=on  BitMask=hex2dec('40000000')  BitMaskRealWorld=Stored Integer
  _Ena : Outport
  _NCR0 : Outport  Port=2
  _Lim+ : Outport  Port=3
  _Lim- : Outport  Port=4
  _OK : Outport  Port=5
  _Icns : Outport  Port=6
  _T-Nlim : Outport  Port=7
  _P-N : Outport  Port=8
  _N-I : Outport  Port=9
  _N0 : Outport  Port=10
  _Rsw : Outport  Port=11
  _Cal0 : Outport  Port=12
  _Cal : Outport  Port=13
  _Tol : Outport  Port=14
  _Rdy : Outport  Port=15
  _Brk : Outport  Port=16
  _SIGNMAG : Outport  Port=17
  _Nclip : Outport  Port=18
  _Nclip+ : Outport  Port=19
  _Nclip- : Outport  Port=20
  _Ird-Dig : Outport  Port=21
  _Ird-rchd : Outport  Port=22
  _Ird-N : Outport  Port=23
  _Ird_TI : Outport  Port=24
  _Ird_TIR : Outport  Port=25
  _2Hz : Outport  Port=26
  _Ird-TM : Outport  Port=27
  _Ird-ANA : Outport  Port=28
  _Iwcns : Outport  Port=29
  _RFE_plus : Outport  Port=30
  _frei : Outport  Port=31
  _Handrad : Outport  Port=32
  wires:
  Ena/1 -> Compare To Zero/1
  NCR0/1 -> Compare To Zero1/1
  Lim+/1 -> Compare To Zero2/1
  Lim-/1 -> Compare To Zero3/1
  OK/1 -> Compare To Zero4/1
  Icns/1 -> Compare To Zero5/1
  T-Nlim/1 -> Compare To Zero6/1
  P-N/1 -> Compare To Zero7/1
  Compare To Zero/1 -> _Ena/1
  Compare To Zero1/1 -> _NCR0/1
  Compare To Zero2/1 -> _Lim+/1
  Compare To Zero3/1 -> _Lim-/1
  Compare To Zero4/1 -> _OK/1
  Compare To Zero5/1 -> _Icns/1
  Compare To Zero6/1 -> _T-Nlim/1
  Compare To Zero7/1 -> _P-N/1
  N-I/1 -> Compare To Zero8/1
  N0/1 -> Compare To Zero9/1
  Rsw/1 -> Compare To Zero10/1
  Cal0/1 -> Compare To Zero11/1
  Cal/1 -> Compare To Zero12/1
  Tol/1 -> Compare To Zero13/1
  Rdy/1 -> Compare To Zero14/1
  Brk/1 -> Compare To Zero15/1
  Compare To Zero8/1 -> _N-I/1
  Compare To Zero9/1 -> _N0/1
  Compare To Zero10/1 -> _Rsw/1
  Compare To Zero11/1 -> _Cal0/1
  Compare To Zero12/1 -> _Cal/1
  Compare To Zero13/1 -> _Tol/1
  Compare To Zero14/1 -> _Rdy/1
  Compare To Zero15/1 -> _Brk/1
  SIGNMAG/1 -> Compare To Zero16/1
  Nclip/1 -> Compare To Zero17/1
  Nclip+/1 -> Compare To Zero18/1
  Nclip-/1 -> Compare To Zero19/1
  Ird-Dig/1 -> Compare To Zero20/1
  Iuse-rchd/1 -> Compare To Zero21/1
  Ird-N/1 -> Compare To Zero22/1
  Ird_TI/1 -> Compare To Zero23/1
  Compare To Zero16/1 -> _SIGNMAG/1
  Compare To Zero17/1 -> _Nclip/1
  Compare To Zero18/1 -> _Nclip+/1
  Compare To Zero19/1 -> _Nclip-/1
  Compare To Zero20/1 -> _Ird-Dig/1
  Compare To Zero21/1 -> _Ird-rchd/1
  Compare To Zero22/1 -> _Ird-N/1
  Compare To Zero23/1 -> _Ird_TI/1
  Ird_TIR/1 -> Compare To Zero24/1
  Compare To Zero24/1 -> _Ird_TIR/1
  Reg 64 Value 0x40/1 -> Data Type Conversion/1
  RFE_plus/1 -> Compare To Zero29/1
  Ird-TM/1 -> Compare To Zero26/1
  frei/1 -> Compare To Zero30/1
  Handrad/1 -> Compare To Zero31/1
  Compare To Zero28/1 -> _Iwcns/1
  Compare To Zero27/1 -> _Ird-ANA/1
  Ird-ANA/1 -> Compare To Zero27/1
  Compare To Zero26/1 -> _Ird-TM/1
  Data Type Conversion/1 -> 2Hz/1, Handrad/1, frei/1, RFE_plus/1, Iwcns/1, Ird-ANA/1, Ird-TM/1, Ird_TIR/1, Nclip/1, Ird_TI/1, Ird-N/1, Iuse-rchd/1, Ird-Dig/1, Nclip-/1, Nclip+/1, SIGNMAG/1, N0/1, Brk/1, Rdy/1, Tol/1, Cal/1, Cal0/1, Rsw/1, N-I/1, NCR0/1, P-N/1, T-Nlim/1, Icns/1, OK/1, Lim-/1, Lim+/1, Ena/1
  Compare To Zero29/1 -> _RFE_plus/1
  Compare To Zero25/1 -> _2Hz/1
  Compare To Zero30/1 -> _frei/1
  Iwcns/1 -> Compare To Zero28/1
  2Hz/1 -> Compare To Zero25/1
  Compare To Zero31/1 -> _Handrad/1
